simulink model "SCARA_SphWrist"  (Simulink 6.5)
settings: Solver=ode45  StartTime=0.0  StopTime=inf  RelTol=1e-3
libraries: vrlib x1
settings Model: Creator=Sohila  LastModifiedBy=Tims
settings OptimizationCC: InitFltsAndDblsToZero=off
settings DebuggingCC: SignalResolutionControl=UseLocalSettings
settings GRTTargetCC: TargetFcnLib=ansi_tfl_table_tmw.mat

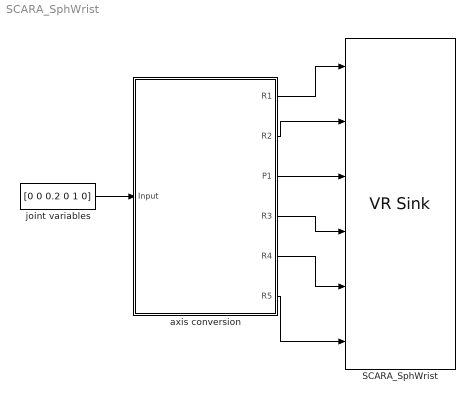
== system SCARA_SphWrist ==
  SCARA_SphWrist : vrlib/VR Sink  SampleTime=0.1  ViewEnable=on  RemoteChange=off  RemoteView=on  FieldsWritten=R1.rotation.4.1.double#R2.rotation.4.1.double#P1.translation.3.1.double#R3.rotation.4.1.double#R4.rotation.4.1.double#R5.rotation.4.1.double  WorldFileName=ScarawithSphericalWrist.WRL  WorldDescription=SCARA Robot Simulation  AutoView=off  FigureProperties="{'Position', 'Name', 'Viewpoint', 'CameraBound', 'CameraDirection', 'CameraPosition', 'CameraUpVector', 'ZoomFactor', 'Antialiasing', 'Headlight', 'Lighting', 'NavPanel', 'StatusBar', 'ToolBar', 'Textures', 'Transparency', 'Wireframe', 'NavZones', 'NavMode', 'NavSpeed', 'Record2DCompressMethod', 'Record2DCompressQuality', 'Record2D', 'Record2DFileName', 'Record2DFPS'; [5.0000000000000000e+000  9.2000000000000000e+001  5.7600000000000000e+002  3.8000000000000000e+002], 'SCARA Robot Simulation ', '_untitled_1', 'on', [0.0000000000000000e+000  0.0000000000000000e+000 -1.0000000000000000e+000], [0.0000000000000000e+000  0.0000000000000000e+000  4.0000000000000000e+000], [0.0000000000000000e+000  1.0000000000000000e+000  0.0000000000000000e+000], [1.0000000000000000e+000], 'off', 'on', 'on', 'halfbar', 'off', 'on', 'on', 'on', 'off', 'off', 'examine', 'normal', 'auto', [7.5000000000000000e+001], 'off', '%f_anim_%n.avi', [1.5000000000000000e+001]}"
  axis conversion : Subsystem
  joint variables : Constant  Value=[0 0 0.2 0 1 0]  OutDataType=fixdt(1, 16)  ConRadixGroup=Use specified scaling  OutScaling=2^0  SampleTime=inf  FramePeriod=inf
  wires:
  joint variables/1 -> axis conversion/1(Input)
  axis conversion/1(R1) -> SCARA_SphWrist/1
  axis conversion/2(R2) -> SCARA_SphWrist/2
  axis conversion/3(P1) -> SCARA_SphWrist/3
  axis conversion/4(R3) -> SCARA_SphWrist/4
  axis conversion/5(R4) -> SCARA_SphWrist/5
  axis conversion/6(R5) -> SCARA_SphWrist/6

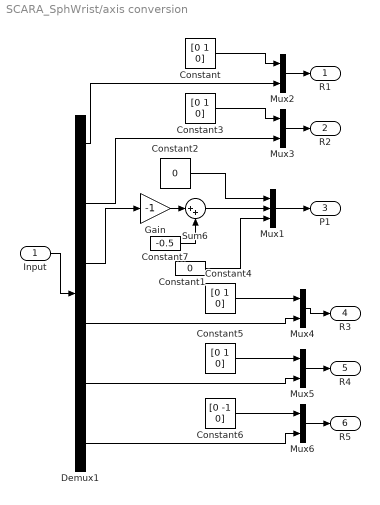
== system SCARA_SphWrist/axis conversion ==
  Input : Inport  OutDataType=fixdt(1,16,0)  OutScaling=[]
  Constant{,3..5} (4 alike) : Constant  Value=[0 1 0]  OutDataType=sfix(16)  ConRadixGroup=Use specified scaling  OutScaling=2^0  SampleTime=inf  FramePeriod=inf
  Constant1 : Constant  Value=0  OutDataType=fixdt(1, 16)  ConRadixGroup=Use specified scaling  OutScaling=2^0  SampleTime=inf  FramePeriod=inf
  Constant2 : Constant  Value=0  OutDataType=fixdt(1, 16)  ConRadixGroup=Use specified scaling  OutScaling=2^0  SampleTime=inf  FramePeriod=inf
  Constant6 : Constant  Value=[0 -1 0]  OutDataType=sfix(16)  ConRadixGroup=Use specified scaling  OutScaling=2^0  SampleTime=inf  FramePeriod=inf
  Constant7 : Constant  Value=-0.5  OutDataType=fixdt(1, 16)  ConRadixGroup=Use specified scaling  OutScaling=2^0  SampleTime=inf  FramePeriod=inf
  Demux1 : Demux  Outputs=6
  Gain : Gain  Gain=-1  ParameterDataType=fixdt(1, 16)  OutDataType=fixdt(1, 16)
  Mux1 : Mux  Inputs=3
  Mux{2..6} (5 alike) : Mux  Inputs=2
  Sum6 : Sum  Inputs=|++  OutDataType=fixdt(1, 16)
  R1 : Outport  OutDataType=fixdt(1,16,0)  OutScaling=[]
  R2 : Outport  Port=2  OutDataType=fixdt(1,16,0)  OutScaling=[]
  P1 : Outport  Port=3  OutDataType=fixdt(1,16,0)  OutScaling=[]
  R3 : Outport  Port=4  OutDataType=fixdt(1,16,0)  OutScaling=[]
  R4 : Outport  Port=5  OutDataType=fixdt(1,16,0)  OutScaling=[]
  R5 : Outport  Port=6  OutDataType=fixdt(1,16,0)  OutScaling=[]
  wires:
  Constant/1 -> Mux2/1
  Constant3/1 -> Mux3/1
  Constant4/1 -> Mux4/1
  Constant5/1 -> Mux5/1
  Constant6/1 -> Mux6/1
  Mux2/1 -> R1/1
  Mux3/1 -> R2/1
  Input/1 -> Demux1/1
  Mux4/1 -> R3/1
  Mux5/1 -> R4/1
  Mux6/1 -> R5/1
  Demux1/1 -> Mux2/2
  Demux1/5 -> Mux5/2
  Gain/1 -> Sum6/1
  Constant7/1 -> Sum6/2
  Mux1/1 -> P1/1
  Constant1/1 -> Mux1/3
  Demux1/2 -> Mux3/2
  Demux1/3 -> Gain/1
  Demux1/4 -> Mux4/2
  Demux1/6 -> Mux6/2
  Constant2/1 -> Mux1/1
  Sum6/1 -> Mux1/2
